simulink model "Control_Matrix"  (R2024b)
settings: Solver=VariableStepAuto  StartTime=0.0  StopTime=10.0  RelTol=1e-3
settings Model: Creator=HP  LastModifiedBy=HP

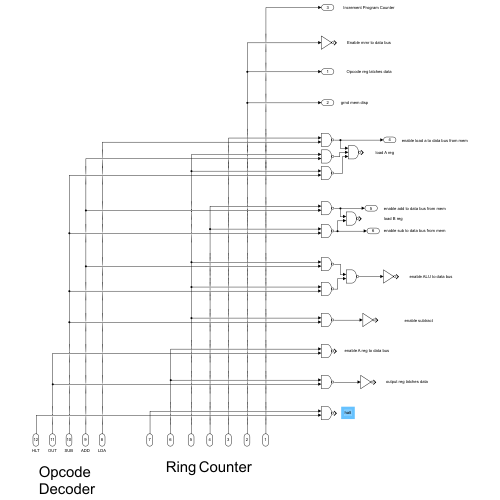
[thumbnail: Simulink's stored preview of the top-level diagram]
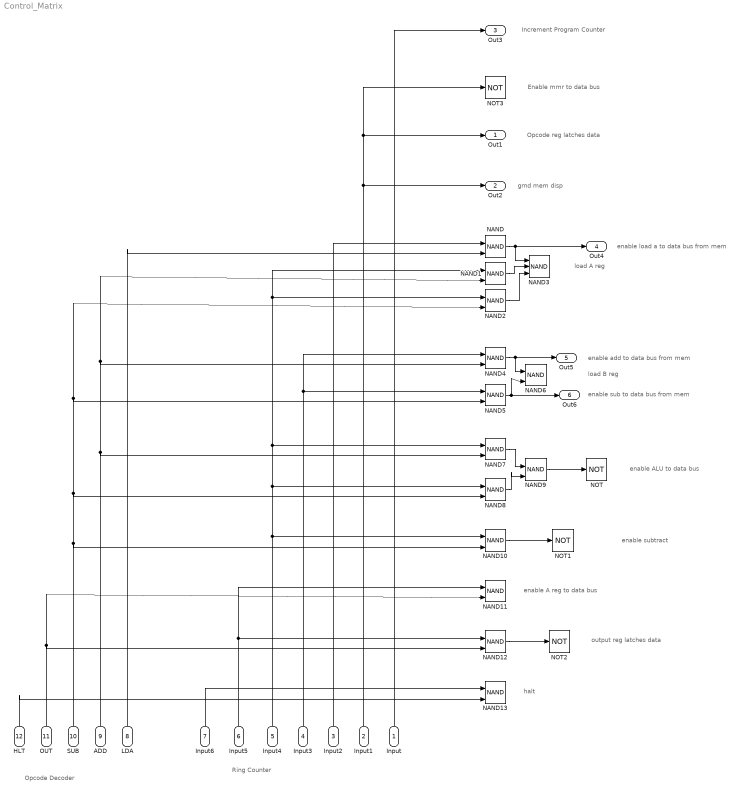
== system Control_Matrix ==
  note: halt
  note: output reg latches data
  note: enable A reg to data bus
  note: enable subtract
  note: enable ALU to data bus
  note: enable add to data bus from mem
  note: load A reg
  note: enable load a to data bus from mem
  note: grnd mem disp
  note: Opcode reg latches data
  note: Enable mmr to data bus
  note: Increment Program Counter
  note: Ring Counter
  note: Opcode Decoder
  note: enable sub to data bus from mem
  note: load B reg
  Input : Inport
  Input1 : Inport  Port=2
  Input2 : Inport  Port=3
  Input3 : Inport  Port=4
  Input4 : Inport  Port=5
  Input5 : Inport  Port=6
  Input6 : Inport  Port=7
  LDA : Inport  Port=8
  ADD : Inport  Port=9
  SUB : Inport  Port=10
  OUT : Inport  Port=11
  HLT : Inport  Port=12
  NAND{,1..2,4..13} (13 alike) : Logic  Operator=NAND  IconShape=distinctive  AllPortsSameDT=off  OutDataTypeStr=boolean
  NAND3 : Logic  Operator=NAND  Inputs=3  IconShape=distinctive  AllPortsSameDT=off  OutDataTypeStr=boolean
  NOT{,1..3} (4 alike) : Logic  Operator=NOT  IconShape=distinctive  AllPortsSameDT=off  OutDataTypeStr=boolean
  Out1 : Outport
  Out2 : Outport  Port=2
  Out3 : Outport  Port=3
  Out4 : Outport  Port=4
  Out5 : Outport  Port=5
  Out6 : Outport  Port=6
  wires:
  NAND/1 -> Out4/1, NAND3/1
  NAND1/1 -> NAND3/2
  NAND2/1 -> NAND3/3
  NAND4/1 -> NAND6/1, Out5/1
  NAND5/1 -> Out6/1, NAND6/2
  NAND7/1 -> NAND9/1
  NAND8/1 -> NAND9/2
  NAND9/1 -> NOT/1
  NAND10/1 -> NOT1/1
  NAND12/1 -> NOT2/1
  Input/1 -> Out3/1
  Input1/1 -> Out2/1, Out1/1, NOT3/1
  Input2/1 -> NAND/1
  LDA/1 -> NAND/2
  Input4/1 -> NAND10/1, NAND8/1, NAND7/1, NAND2/1, NAND1/1
  ADD/1 -> NAND7/2, NAND4/2, NAND1/2
  SUB/1 -> NAND10/2, NAND8/2, NAND5/2, NAND2/2
  Input3/1 -> NAND5/1, NAND4/1
  Input5/1 -> NAND12/1, NAND11/1
  OUT/1 -> NAND12/2, NAND11/2
  Input6/1 -> NAND13/1
  HLT/1 -> NAND13/2
